simulink model "untitled"  (R2019b)
settings: Solver=VariableStepAuto  StartTime=0.0  StopTime=3200  RelTol=1e-3  EnableMultiTasking=on
values from neighbouring files (symbols this model uses):
  T_b = 2    [constants.m]    (also in main.m)
libraries: simulink x3, commrandsrc3 x1, commutil2 x1, commfilt2 x1
settings Model: Creator=Elena  LastModifiedBy=Elena

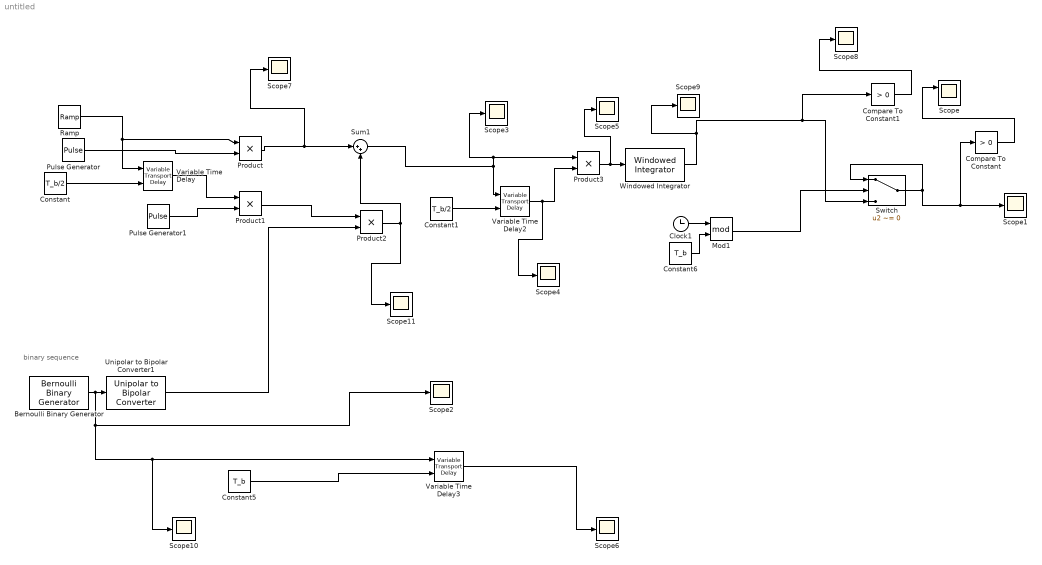
== system untitled ==
  note: binary sequence
  Bernoulli Binary Generator : commrandsrc3/Bernoulli Binary Generator  ProbabilityOfZero=0.5  SeedSource=Auto  Seed=0  SampleTime=T_b  SamplesPerFrame=1  OutputDataType=double  SimulateUsing=Interpreted execution
      settings: SourceProductName=Communications Toolbox
  Clock1 : Clock
  Compare To Constant : simulink/Logic and Bit Operations/Compare To Constant  relop=>  const=0  OutDataTypeStr=boolean
  Compare To Constant1 : simulink/Logic and Bit Operations/Compare To Constant  relop=>  const=0  OutDataTypeStr=boolean
  Constant : Constant  Value=T_b/2
  Constant1 : Constant  Value=T_b/2
  Constant5 : Constant  Value=T_b
  Constant6 : Constant  Value=T_b
  Mod1 : Math  Operator=mod  SignedPower=off  SaturateOnIntegerOverflow=on
  Product{,1..3} (4 alike) : Product
  Pulse Generator : DiscretePulseGenerator  PulseType=Time based  Period=T_b  PulseWidth=50
  Pulse Generator1 : DiscretePulseGenerator  PulseType=Time based  Period=T_b  PulseWidth=50  PhaseDelay=T_b/2
  Ramp : simulink/Sources/Ramp  slope=1  start=0  InitialOutput=0
  Scope : Scope  NumInputPorts=2
  Scope{1..11} (11 alike) : Scope
  Sum1 : Sum  Inputs=|++
  Switch : Switch  Criteria=u2 ~= 0
  Unipolar to Bipolar Converter1 : commutil2/Unipolar to Bipolar Converter  M=2  polarity=Positive  dataType=Inherit via internal rule
      settings: SourceProductName=Communications Toolbox
  Variable Time Delay : VariableTransportDelay  MaximumDelay=100
  Variable Time Delay2 : VariableTransportDelay  MaximumDelay=1000
  Variable Time Delay3 : VariableTransportDelay  MaximumDelay=100
  Windowed Integrator : commfilt2/Windowed Integrator  integperiod=T_b/2  InputProcessing=Columns as channels (frame based)  roundingMode=Floor  overflowMode=off  coeffDataTypeStr=Inherit: Same word length as input  coeffMin=[]  coeffMax=[]  coeffLastDataTypeStr=Inherit: Same word length as input  accumDataTypeStr=Inherit: Same as product output  accumLastDataTypeStr=Inherit: Same as product output  outputDataTypeStr=Inherit: Same as accumulator  outputMin=[]  outputMax=[]  outputLastDataTypeStr=Inherit: Same as accumulator
      settings: SourceProductName=Communications Toolbox  SourceProductBaseCode=CM
  wires:
  Product2/1 -> Sum1/2, Scope11/1
  Bernoulli Binary Generator/1 -> Scope2/1, Scope10/1, Variable Time Delay3/1, Unipolar to Bipolar Converter1/1
  Product/1 -> Scope7/1, Sum1/1
  Pulse Generator/1 -> Product/2
  Product1/1 -> Product2/1
  Ramp/1 -> Variable Time Delay/1, Product/1
  Constant/1 -> Variable Time Delay/2
  Pulse Generator1/1 -> Product1/2
  Variable Time Delay/1 -> Product1/1
  Unipolar to Bipolar Converter1/1 -> Product2/2
  Variable Time Delay2/1 -> Scope4/1, Product3/2
  Constant1/1 -> Variable Time Delay2/2
  Product3/1 -> Scope5/1, Windowed Integrator/1
  Sum1/1 -> Product3/1, Scope3/1, Variable Time Delay2/1
  Constant5/1 -> Variable Time Delay3/2
  Variable Time Delay3/1 -> Scope6/1
  Compare To Constant/1 -> Scope/1
  Mod1/1 -> Switch/2
  Constant6/1 -> Mod1/2
  Clock1/1 -> Mod1/1
  Switch/1 -> Switch/1, Compare To Constant/1, Scope1/1
  Windowed Integrator/1 -> Scope9/1, Compare To Constant1/1, Switch/3
  Compare To Constant1/1 -> Scope8/1
